simulink model "BergmanModelExtendedv2"  (R2021a)
settings: Solver=VariableStepAuto  StartTime=0.0  StopTime=1000  RelTol=1e-3
model workspace (MAT data in the model file):
  Gb = 100
  Ib = 0.2
  U1 = 0
  U2 = 0
  U3 = 0
  VolG = 117
  W = 70
  a1 = 0.00158
  a2 = 0.056
  a3 = 0.00195
  a4 = 0.0485
  a5 = 0.00125
  a6 = 0.075
  n = 0.142
  p1 = 0.035
  p2 = 0.05
  p3 = 2.8e-05
  p4 = 0.098
settings Model: Creator=marti  LastModifiedBy=13234
settings SolverCC: AlgebraicLoopSolver=TrustRegion
settings DataIOCC: ReturnWorkspaceOutputs=off
settings DebuggingCC: SFMachineParentedDataDiag=warning  ArithmeticOperatorsInVariantConditions=warning
settings SFSimCC: CustomCodeUndefinedFunction=UseInterfaceOnly

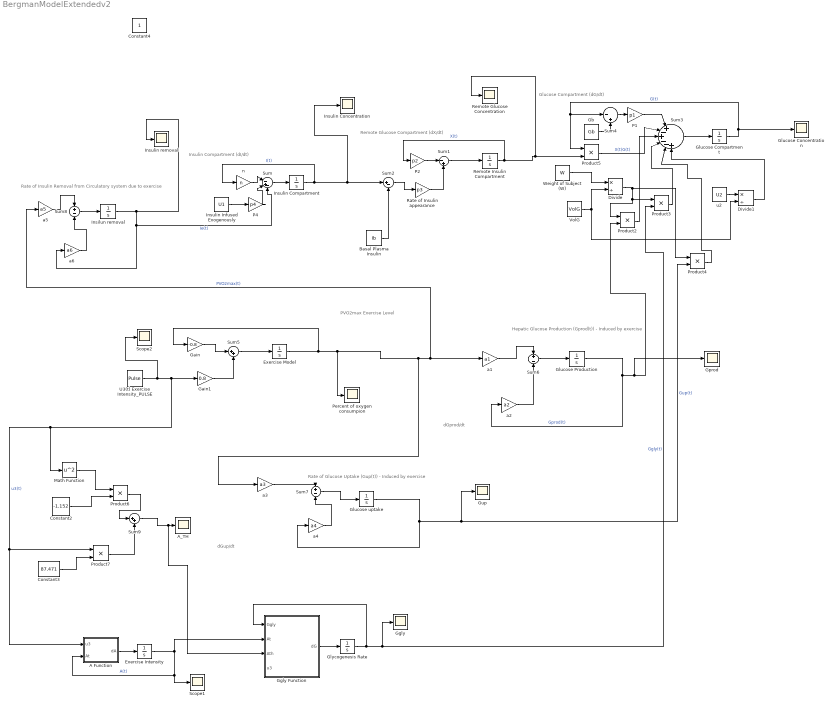
== system BergmanModelExtendedv2 ==
  note: dGprod/dt
  note: dGup/dt
  note: Rate of Insulin Removal from Circulatory system due to exercise
  note: Rate of Glucose Uptake (Gup(t)) - Induced by exercise
  note: Hepatic Glucose Production (Gprod(t)) - Induced by exercise
  note: PVO2max Exercise Level
  note: Insulin Compartment (dI/dt)
  note: Glucose Compartment (dG/dt)
  note: Remote Glucose Compartment (dX/dt)
  A Function : MATLAB Function  TreatAsAtomicUnit=on
  A_TH : Scope
  "Basal Plasma Insulin " : Constant  Value=Ib  VectorParams1D=off
  Constant2 : Constant  Value=-1.152
  Constant3 : Constant  Value=87.471
  Divide : Product  Inputs=*/
  Divide1 : Product  Inputs=*/
  Exercise Intensity : Integrator
  "Exercise Model " : Integrator
  Gain : Gain  Gain=-0.8
  Gain1 : Gain  Gain=0.8
  Gb : Constant  Value=Gb
  Ggly : Scope
  Ggly Function : MATLAB Function  TreatAsAtomicUnit=on
  Glucose Compartment : Integrator  InitialCondition=Gb
  Glucose Concentration : Scope
  Glucose Production : Integrator
  Glucose uptake : Integrator
  Glycogenesis Rate : Integrator
  Gprod : Scope
  Gup : Scope
  Insilun removal : Integrator
  Insulin Compartment : Integrator  InitialCondition=1
  Insulin Concentration : Scope
  Insulin Infused Exogenously : Constant  Value=U1  OutMin=0  OutMax=100
  "Insulin removal " : Scope
  Math Function : Math  Operator=square  SaturateOnIntegerOverflow=on
  P1 : Gain  Gain=p1
  P2 : Gain  Gain=p2
  P4 : Gain  Gain=p4
  "Percent of oxygen consumpion " : Scope
  Product{2..7} (6 alike) : Product
  "Rate of Insulin appearance " : Gain  Gain=p3
  Remote Glucose Concentration : Scope
  Remote Insulin Compartment : Integrator
  Scope1 : Scope
  Scope2 : Scope
  Sum : Sum  Inputs=|-+-
  Sum1 : Sum  Inputs=|-+
  Sum2 : Sum  Inputs=|+-
  Sum3 : Sum  Inputs=|+-+--+
  Sum4 : Sum  Inputs=|-+
  Sum5 : Sum  Inputs=|++
  Sum6 : Sum  Inputs=+-
  Sum7 : Sum  Inputs=+-
  Sum8 : Sum  Inputs=+-
  Sum9 : Sum  Inputs=|++
  U3(t) Exercise Intensity_PULSE : DiscretePulseGenerator  PulseType=Time based  Amplitude=U3  Period=500  PulseWidth=20  PhaseDelay=100
  VolG : Constant  Value=VolG
  Weight of Subject (W) : Constant  Value=W
  a1 : Gain  Gain=a1
  a2 : Gain  Gain=a2
  a3 : Gain  Gain=a3
  a4 : Gain  Gain=a4
  a5 : Gain  Gain=a5
  a6 : Gain  Gain=a6
  n : Gain  Gain=n
  u2 : Constant  Value=U2
  Constant4 : Constant  IOType=siggen
  wires:
  Remote Insulin Compartment/1 -> P2/1, Product5/2, Remote Glucose Concentration/1  "X(t)"
  Insulin Compartment/1 -> n/1, Insulin Concentration/1, Sum2/1  "I(t)"
  Product5/1 -> Sum3/2  "X(t)G(t)"
  "Rate of Insulin appearance "/1 -> Sum1/2
  Sum1/1 -> Remote Insulin Compartment/1
  Gb/1 -> Sum4/2
  Sum/1 -> Insulin Compartment/1
  P2/1 -> Sum1/1
  Sum3/1 -> Glucose Compartment/1
  P1/1 -> Sum3/1
  Sum4/1 -> P1/1
  Glucose Compartment/1 -> Product5/1, Sum4/1, Glucose Concentration/1  "G(t)"
  Sum2/1 -> "Rate of Insulin appearance "/1
  Sum5/1 -> "Exercise Model "/1
  n/1 -> Sum/1
  P4/1 -> Sum/2
  "Basal Plasma Insulin "/1 -> Sum2/2
  "Exercise Model "/1 -> Gain/1, "Percent of oxygen consumpion "/1, a3/1, a5/1, a1/1  "PVO2max(t)"
  a1/1 -> Sum6/1
  Sum6/1 -> Glucose Production/1
  a2/1 -> Sum6/2
  Glucose Production/1 -> Gprod/1, Product2/2, a2/1  "Gprod(t)"
  a3/1 -> Sum7/1
  Sum7/1 -> Glucose uptake/1
  Glucose uptake/1 -> Gup/1, Product4/2, a4/1  "Gup(t)"
  a4/1 -> Sum7/2
  a5/1 -> Sum8/1
  Sum8/1 -> Insilun removal/1
  Insilun removal/1 -> a6/1, Sum/3, "Insulin removal "/1  "Ie(t)"
  a6/1 -> Sum8/2
  Weight of Subject (W)/1 -> Divide/1
  VolG/1 -> Divide/2, Divide1/2
  Divide/1 -> Product3/1, Product2/1, Product4/1
  u2/1 -> Divide1/1
  Product2/1 -> Sum3/3
  Product3/1 -> Sum3/4
  Product4/1 -> Sum3/5
  Divide1/1 -> Sum3/6
  Insulin Infused Exogenously/1 -> P4/1
  Product6/1 -> Sum9/1
  Constant2/1 -> Product6/2
  Sum9/1 -> Ggly Function/3(Ath), A_TH/1
  Math Function/1 -> Product6/1
  Constant3/1 -> Product7/2
  Product7/1 -> Sum9/2
  A Function/1(dA) -> Exercise Intensity/1
  Exercise Intensity/1 -> Scope1/1, A Function/2(At), Ggly Function/2(At)  "A(t)"
  Ggly Function/1(dG) -> Glycogenesis Rate/1
  Glycogenesis Rate/1 -> Ggly Function/1(Ggly), Ggly/1, Product3/2  "Ggly(t)"
  Gain/1 -> Sum5/1
  Gain1/1 -> Sum5/2
  U3(t) Exercise Intensity_PULSE/1 -> Scope2/1, A Function/1(u3), Product7/1, Math Function/1, Gain1/1  "u3(t)"

== matlab function BergmanModelExtendedv2/A Function ==
  data: u3 input; dA output; At input
function dA = fcn(u3, At)
    if u3 == 0
        dA = -(At/0.001);
        return
    else
        dA = u3;
        return
    end

== matlab function BergmanModelExtendedv2/Ggly Function ==
  data: dG output; Ggly input; At input; Ath input; u3 input
function dG = Ggly(Ggly, At, Ath, u3)
k = 0.0108;
T1 = 6;
dG = 0;
    if u3 == 0
        dG = -(Ggly/T1);
        return
    end
    if At < Ath
        dG = 0;
        return
    end
    if At >= Ath
        dG = k;
        return
    end
